simulink model "pendulum_adaptive_feedback_linearization"  (R2023a)
settings: Solver=FixedStepAuto  StartTime=0.0  StopTime=200.0  FixedStep=0.01  RelTol=1e-3
settings Model: Creator=Mmoha  LastModifiedBy=Mmoha

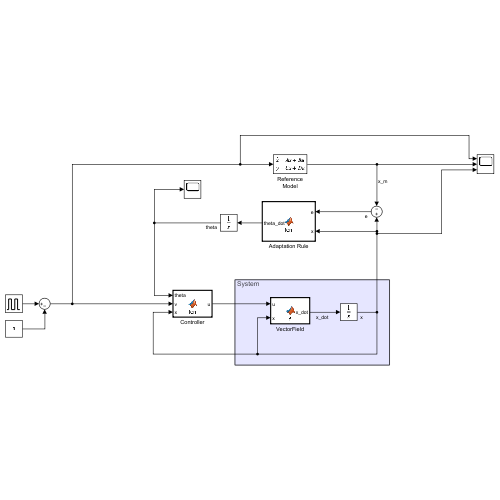
[thumbnail: Simulink's stored preview of the top-level diagram]
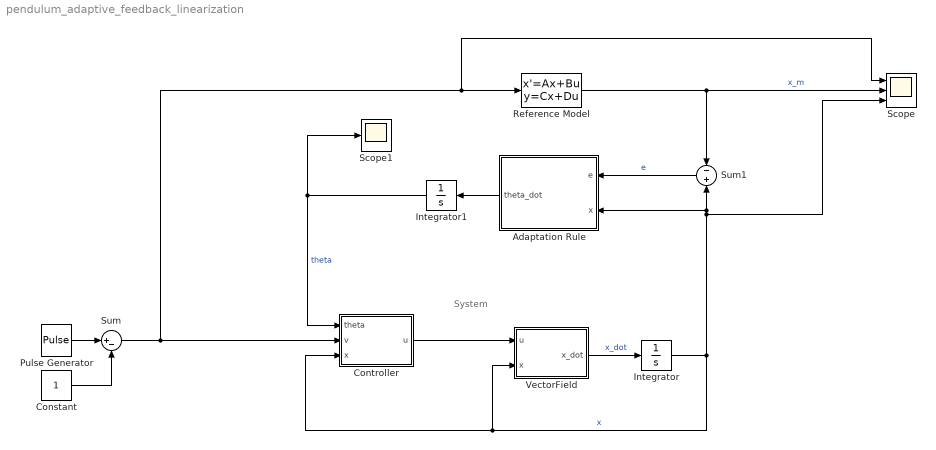
== system pendulum_adaptive_feedback_linearization ==
  note: System
  Adaptation Rule : MATLAB Function  TreatAsAtomicUnit=on
  Constant : Constant
  Controller : MATLAB Function  TreatAsAtomicUnit=on
  Integrator : Integrator  InitialCondition=[1; 0]
  Integrator1 : Integrator
  Pulse Generator : DiscretePulseGenerator  PulseType=Time based  Amplitude=2  Period=50  PulseWidth=50
  Reference Model : StateSpace  A=[0, 1; -1 -2]  B=[0; 1]  C=eye(2)  D=[0; 0]  InitialCondition=[1; 0]
  Scope : Scope  NumInputPorts=3
  Scope1 : Scope
  Sum : Sum  Inputs=|+-
  Sum1 : Sum  Inputs=-|+
  VectorField : MATLAB Function  TreatAsAtomicUnit=on
  wires:
  VectorField/1(x_dot) -> Integrator/1  "x_dot"
  Integrator/1 -> Adaptation Rule/2(x), Sum1/2, Scope/3, Controller/3(x), VectorField/2(x)  "x"
  Sum/1 -> Scope/1, Reference Model/1, Controller/2(v)
  Reference Model/1 -> Sum1/1, Scope/2  "x_m"
  Pulse Generator/1 -> Sum/1
  Constant/1 -> Sum/2
  Sum1/1 -> Adaptation Rule/1(e)  "e"
  Adaptation Rule/1(theta_dot) -> Integrator1/1
  Integrator1/1 -> Scope1/1, Controller/1(theta)  "theta"
  Controller/1(u) -> VectorField/1(u)

== matlab function pendulum_adaptive_feedback_linearization/VectorField ==
  data: u input size=1; x_dot output size=[2 1]; x input size=[2 1]
function x_dot = f(u,x)

x_dot = [
    x(2); 
    -sin(x(1))-x(2)+1+0.5*u
    ];

== matlab function pendulum_adaptive_feedback_linearization/Adaptation Rule ==
  data: e input; theta_dot output; x input
function theta_dot = fcn(e,x)

gamma = 1;

Psi = [
    0, 0,    0,    0;
    1, x(1), x(2), sin(x(1))
    ];

P = [1.5, 0.5; 0.5, 0.5];

theta_dot = -gamma * Psi' * P * e;

== matlab function pendulum_adaptive_feedback_linearization/Controller ==
  data: theta input; v input; u output; x input
function u = fcn(theta, v,x)

Psi = [1, x(1), x(2), sin(x(1))];

u = -x(1) -2*x(2) + Psi*theta + v;
